simulink model "ClosedLoopStimXpcTarget"  (R2016b)
settings: Solver=FixedStepDiscrete  StartTime=0.0  StopTime=inf  FixedStep=sCoreParams.core.stepPeriod  RelTol=1e-3  EnableMultiTasking=on
values from neighbouring files (symbols this model uses):
  sCoreParams = InitCoreParams_Dependent(sCoreParams)    [initializationScript.m]
settings Model: DataTypeOverride=Double  MinMaxOverflowLogging=ForceOff  Creator=rzelmann  LastModifiedBy=rzelmann
settings SolverCC: EnableConcurrentExecution=on  ConcurrentTasks=on
settings DataIOCC: SaveFormat=StructureWithTime
settings OptimizationCC: DefaultParameterBehavior=Inlined  EfficientFloat2IntCast=on  LifeSpan=inf
settings DebuggingCC: UniqueDataStoreMsg=error  StrictBusMsg=ErrorOnBusTreatedAsVector  SFUnexpectedBacktrackingDiag=warning  SFNoUnconditionalDefaultTransitionDiag=warning  SFExecutionAtInitializationDiag=none
settings HardwareCC: ProdBitPerPointer=32  ProdBitPerSizeT=32  ProdBitPerPtrDiffT=32  ProdLargestAtomicFloat=None  ProdWordSize=32  ProdLongLongMode=on  ProdHWDeviceType=Generic->32-bit x86 compatible
settings ModelReferenceCC: ModelReferenceNumInstancesAllowed=Single
settings RTWCC: SystemTargetFile=slrt.tlc  TLCOptions="-axPCMaxOverloads=30            -axPCOverLoadLen=2 -axPCStartupFlag=5"  TemplateMakefile=slrt_default_tmf  Description=Simulink Real-Time  RTWCompilerOptimization=on
settings CodeAppCC: MaxIdLength=63
settings ConfigComp: CovMetricSettings=dw  CovHtmlReporting=on  CovSaveCumulativeToWorkspaceVar=on  CovSaveSingleToWorkspaceVar=on  CovExternalEMLEnable=off

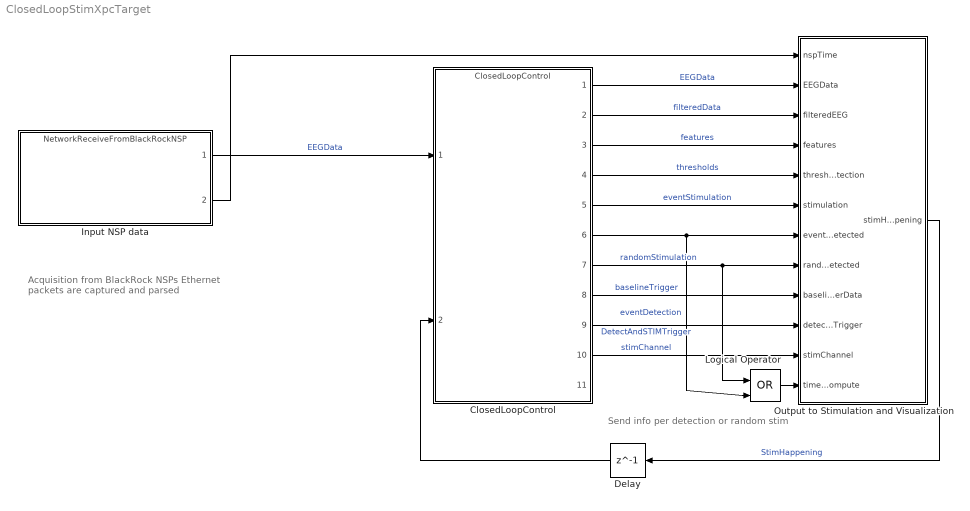
== system ClosedLoopStimXpcTarget ==
  note: Acquisition from BlackRock NSPs
      | Ethernet packets are captured and parsed
  note: Send info per detection or random stim
  ClosedLoopControl : ModelReference  ModelNameDialog=ClosedLoopControl  SimulationMode=Normal  ModelReferenceVersion=1.722
  Delay : Delay  DelayLength=1  InitialCondition=0  InputProcessing=Columns as channels (frame based)  SampleTime=sCoreParams.core.stepPeriod
  Input NSP data : ModelReference  ModelNameDialog=NetworkReceiveFromBlackRockNSP.slx  SimulationMode=Normal  ModelReferenceVersion=1.231
  Logical Operator : Logic  Operator=OR  IconShape=distinctive  AllPortsSameDT=off  OutDataTypeStr=boolean
  Output to Stimulation and Visualization : Subsystem
  wires:
  Output to Stimulation and Visualization/1(stimHappening) -> Delay/1  "StimHappening"
  Input NSP data/1 -> ClosedLoopControl/1  "EEGData"
  ClosedLoopControl/1 -> Output to Stimulation and Visualization/2(EEGData)  "EEGData"
  Input NSP data/2 -> Output to Stimulation and Visualization/1(nspTime)
  ClosedLoopControl/4 -> Output to Stimulation and Visualization/5(thresholdUsedInDetection)  "thresholds"
  ClosedLoopControl/6 -> Logical Operator/2, Output to Stimulation and Visualization/7(eventDetected)  "eventDetection"
  ClosedLoopControl/8 -> Output to Stimulation and Visualization/9(baselineTriggerData)  "baselineTrigger"
  ClosedLoopControl/9 -> Output to Stimulation and Visualization/10(detectStimTrigger)  "DetectAndSTIMTrigger"
  ClosedLoopControl/10 -> Output to Stimulation and Visualization/11(stimChannel)  "stimChannel"
  Delay/1 -> ClosedLoopControl/2
  ClosedLoopControl/7 -> Logical Operator/1, Output to Stimulation and Visualization/8(randomDetected)  "randomStimulation"
  ClosedLoopControl/5 -> Output to Stimulation and Visualization/6(stimulation)  "eventStimulation"
  ClosedLoopControl/3 -> Output to Stimulation and Visualization/4(features)  "features"
  ClosedLoopControl/2 -> Output to Stimulation and Visualization/3(filteredEEG)  "filteredData"
  Logical Operator/1 -> Output to Stimulation and Visualization/12(timeToCompute)

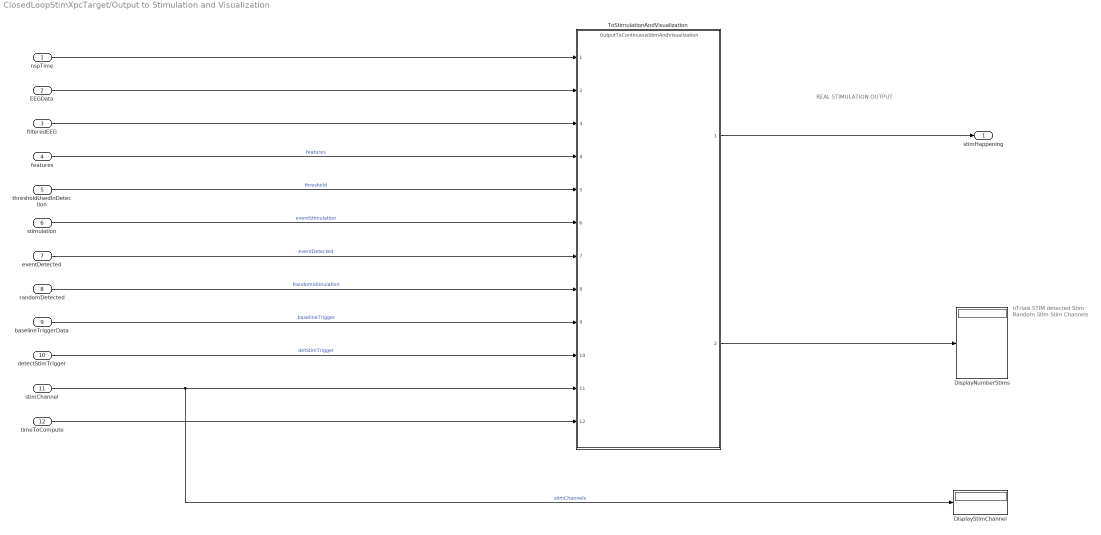
== system ClosedLoopStimXpcTarget/Output to Stimulation and Visualization ==
  note: nTrials
      | STIM
      | detected Stim
      | Random Stim
      | Stim Channels
  note: REAL STIMULATION OUTPUT
  nspTime : Inport
  EEGData : Inport  Port=2
  filteredEEG : Inport  Port=3
  features : Inport  Port=4
  thresholdUsedInDetection : Inport  Port=5
  stimulation : Inport  Port=6
  eventDetected : Inport  Port=7
  randomDetected : Inport  Port=8
  baselineTriggerData : Inport  Port=9  OutDataTypeStr=int32
  detectStimTrigger : Inport  Port=10  OutDataTypeStr=int32
  stimChannel : Inport  Port=11
  timeToCompute : Inport  Port=12  OutDataTypeStr=boolean
  DisplayNumberStims : Display
      settings: Format=decimal (Stored Integer)
  DisplayStimChannel : Display
  ToStimulationAndVisualization : ModelReference  ModelNameDialog=OutputToContinuousStimAndVisualization.slx  SimulationMode=Normal  ModelReferenceVersion=1.314
  stimHappening : Outport  OutDataTypeStr=boolean  SampleTime=sCoreParams.core.stepPeriod
  wires:
  stimChannel/1 -> ToStimulationAndVisualization/11, DisplayStimChannel/1  "stimChannels"
  ToStimulationAndVisualization/2 -> DisplayNumberStims/1
  ToStimulationAndVisualization/1 -> stimHappening/1
  nspTime/1 -> ToStimulationAndVisualization/1
  EEGData/1 -> ToStimulationAndVisualization/2
  filteredEEG/1 -> ToStimulationAndVisualization/3
  features/1 -> ToStimulationAndVisualization/4  "features"
  thresholdUsedInDetection/1 -> ToStimulationAndVisualization/5  "threshold"
  stimulation/1 -> ToStimulationAndVisualization/6  "eventStimulation"
  detectStimTrigger/1 -> ToStimulationAndVisualization/10  "detStimTrigger"
  baselineTriggerData/1 -> ToStimulationAndVisualization/9  "baselineTrigger"
  timeToCompute/1 -> ToStimulationAndVisualization/12
  eventDetected/1 -> ToStimulationAndVisualization/7  "eventDetected"
  randomDetected/1 -> ToStimulationAndVisualization/8  "RandomStimulation"
